simulink model "frame_1"  (Simulink 7.8)
settings: Solver=FixedStepDiscrete  StartTime=0.0  StopTime=1  MaxStep=1e-4  RelTol=1e-3
undefined symbols (not defined in the file or in its folder): get
libraries: dsparch4 x1, dspsigops x1, dspsnks4 x1
settings Model: Creator=svenhoffmann  LastModifiedBy=josef  ExtModeAutoUpdateStatusClock=off
settings DataIOCC: SaveFormat=StructureWithTime
settings OptimizationCC: InlineInvariantSignals=on  InitFltsAndDblsToZero=on
settings DebuggingCC: SaveWithParameterizedLinksMsg=none  SignalResolutionControl=TryResolveAllWithWarning  MultiTaskDSMMsg=warning  MultiTaskCondExecSysMsg=none  FcnCallInpInsideContextMsg=Use local settings  StrictBusMsg=None
settings RTWCC: IncludeERTFirstTime=on
settings GRTTargetCC: TargetFcnLib=ansi_tfl_tmw.mat

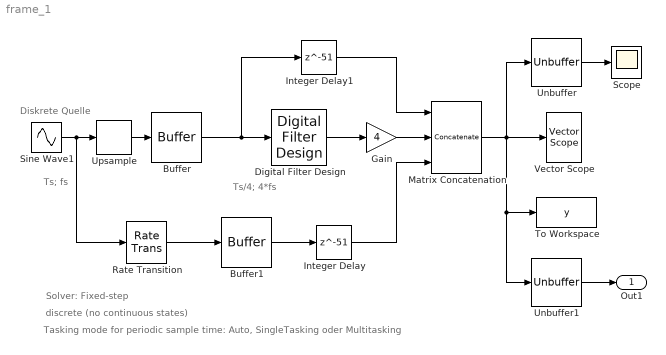
== system frame_1 ==
  note: Solver: Fixed-step
  note: discrete (no continuous states)
  note: Tasking mode for periodic sample time: Auto, SingleTasking oder Multitasking
  note: Diskrete Quelle
  note: Ts; fs
  note: Ts/4; 4*fs
  Buffer : Buffer  N=256
  Buffer1 : Buffer  N=256
  Digital Filter Design : dsparch4/Digital Filter Design  mwdsp_browser_bugfix_var=off
  Gain : Gain  Gain=4
  Integer Delay : Delay  DelayLength=51  InputProcessing=Inherited
  Integer Delay1 : Delay  DelayLength=51  InputProcessing=Inherited
  Matrix Concatenation : Concatenate  NumInputs=3  Mode=Multidimensional array  ConcatenateDimension=2
  Rate Transition : RateTransition
  Scope : Scope
  Sine Wave1 : Sin  Frequency=2*pi*100  SampleTime=1/1000
  To Workspace : ToWorkspace  VariableName=y  SampleTime=-1  SaveFormat=Structure
  Unbuffer : Unbuffer
  Unbuffer1 : Unbuffer
  Upsample : dspsigops/Upsample  N=4  phase=0  InputProcessing=Inherited (this choice will be removed - see release notes)  RateOptions=Allow multirate processing  ic=0  mode=Unused parameter value
  Vector Scope : dspsnks4/Vector Scope  ScopeProperties=on  Domain=Time  HorizSpan=1  DisplayProperties=off  AxisGrid=on  Memory=off  FrameNumber=on  AxisLegend=off  AxisZoom=off  OpenScopeAtSimStart=on  OpenScopeImmediately=off  FigPos=get(0,'defaultfigureposition')  AxisProperties=off  XUnits=Hertz  XRange=[0...Fs/2]  InheritXIncr=on  XIncr=1  XLabel=Time  XLimit=Auto  XMin=0  XMax=1  XStart=0  YUnits=dB  YLabel=Amplitude  LineProperties=off  XAxisParamsVer=6.8
      settings: YMin=-0.998609342109915  YMax=0.998609342109915
  Out1 : Outport
  wires:
  Sine Wave1/1 -> Upsample/1, Rate Transition/1
  Upsample/1 -> Buffer/1
  Digital Filter Design/1 -> Gain/1
  Integer Delay/1 -> Matrix Concatenation/3
  Buffer/1 -> Integer Delay1/1, Digital Filter Design/1
  Gain/1 -> Matrix Concatenation/2
  Integer Delay1/1 -> Matrix Concatenation/1
  Matrix Concatenation/1 -> Vector Scope/1, Unbuffer/1, To Workspace/1, Unbuffer1/1
  Buffer1/1 -> Integer Delay/1
  Unbuffer/1 -> Scope/1
  Unbuffer1/1 -> Out1/1
  Rate Transition/1 -> Buffer1/1
